simulink subsystem "Direct_Z_Position_Command"  (R2023a)
settings: Solver=VariableStepAuto  StartTime=0.0  StopTime=10.0  RelTol=1e-3
undefined symbols (not defined in the file or in its folder): flight_mode
libraries: eeGeneralControl x2, simulink x1
settings Model: Creator=thesa  LastModifiedBy=thesa

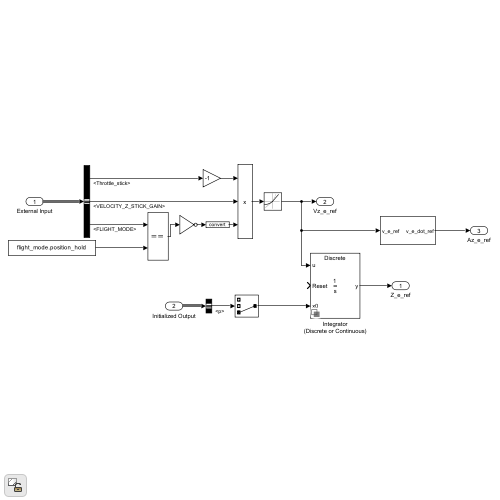
[thumbnail: Simulink's stored preview of the top-level diagram]
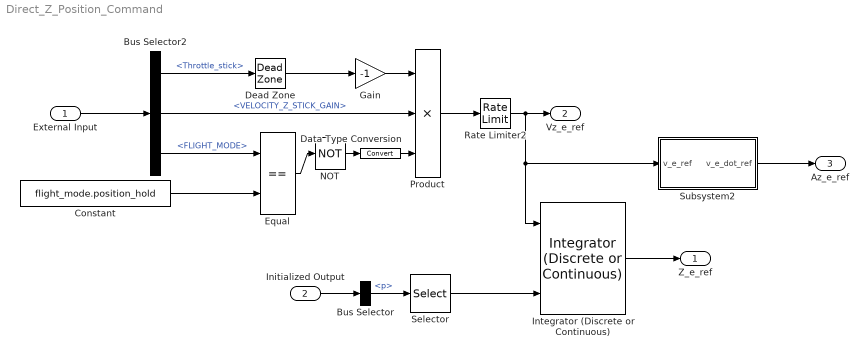
== system Direct_Z_Position_Command ==
  External Input : Inport
  Initialized Output : Inport  Port=2
  Bus Selector : BusSelector  OutputSignals=References.trajectory.p
  Bus Selector2 : BusSelector  OutputSignals=Pilot Input.Sticks.Throttle_stick,Pilot Input.Parameters.VELOCITY_Z_STICK_GAIN,Pilot Input.FLIGHT_MODE
  Constant : Constant  Value=flight_mode.position_hold
  Data Type Conversion : DataTypeConversion  SaturateOnIntegerOverflow=off  RndMeth=Floor
  Dead Zone : DeadZone  LowerValue=-0.15  UpperValue=0.15
  Equal : RelationalOperator  Operator===  OutDataTypeStr=boolean  RndMeth=Simplest  InputSameDT=off
  Gain : Gain  Gain=-1
  Integrator (Discrete or Continuous) : eeGeneralControl/Integrator (Discrete or Continuous)  LabelModeActiveChoice=Discrete  ExternalReset=either  LimitType=Anti-windup  B=inf  A=-inf  Ts=-1
      settings: LibrarySourceBlock=|
      | ee_sl_lib/General Control/Integrator
      | (Discrete or Continuous)
  NOT : Logic  Operator=NOT  IconShape=distinctive  AllPortsSameDT=off  OutDataTypeStr=boolean
  Product : Product  Inputs=3
  Rate Limiter2 : RateLimiter  RisingSlewLimit=0.8  FallingSlewLimit=-0.8  SampleTimeMode=inherited
  Selector : Selector  InputPortWidth=3  IndexOptions=Index vector (dialog)  Indices=[3]  OutputSizes=1
  Subsystem2 : Subsystem
  Z_e_ref : Outport
  Vz_e_ref : Outport  Port=2
  Az_e_ref : Outport  Port=3
  wires:
  External Input/1 -> Bus Selector2/1
  Product/1 -> Rate Limiter2/1
  Bus Selector2/1 -> Dead Zone/1  "<Throttle_stick>"
  Bus Selector2/2 -> Product/2  "<VELOCITY_Z_STICK_GAIN>"
  Gain/1 -> Product/1
  Rate Limiter2/1 -> Vz_e_ref/1, Integrator (Discrete or Continuous)/1, Subsystem2/1(v_e_ref)
  Initialized Output/1 -> Bus Selector/1
  Bus Selector/1 -> Selector/1  "<p>"
  Subsystem2/1(v_e_dot_ref) -> Az_e_ref/1
  Integrator (Discrete or Continuous)/1 -> Z_e_ref/1
  Selector/1 -> Integrator (Discrete or Continuous)/3
  Equal/1 -> NOT/1
  NOT/1 -> Data Type Conversion/1
  Data Type Conversion/1 -> Product/3
  Bus Selector2/3 -> Equal/1  "<FLIGHT_MODE>"
  Constant/1 -> Equal/2
  Dead Zone/1 -> Gain/1

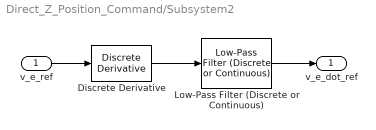
== system Direct_Z_Position_Command/Subsystem2 ==
  v_e_ref : Inport
  Discrete Derivative : simulink/Discrete/Discrete Derivative  gainval=1.0  ICPrevScaledInput=0.0  OutMin=[]  OutMax=[]  OutDataType=fixdt(1, 16)  OutScaling=2^-10  DoSatur=off
  Low-Pass Filter (Discrete or Continuous) : eeGeneralControl/Low-Pass Filter (Discrete or Continuous)  K=1  T=1/2  B=inf  A=-inf  init_option=Inherited from block input  x0=0  Ts=-1
  v_e_dot_ref : Outport
  wires:
  Discrete Derivative/1 -> Low-Pass Filter (Discrete or Continuous)/1
  v_e_ref/1 -> Discrete Derivative/1
  Low-Pass Filter (Discrete or Continuous)/1 -> v_e_dot_ref/1
